simulink model "last_pressed_led"  (R2025a)
settings: Solver=FixedStepDiscrete  StartTime=0.0  StopTime=10  FixedStep=1  RelTol=1e-3
settings Model: Creator=mahij  LastModifiedBy=mahij

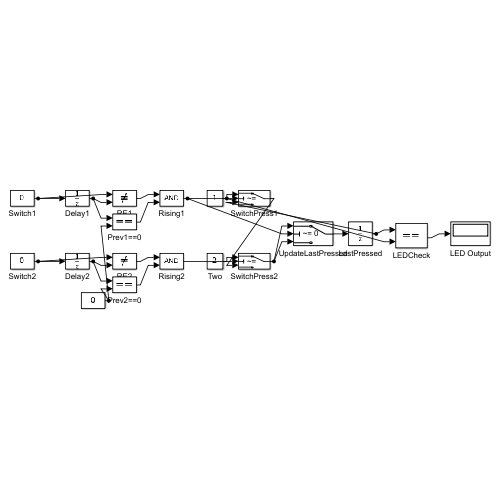
[thumbnail: Simulink's stored preview of the top-level diagram]
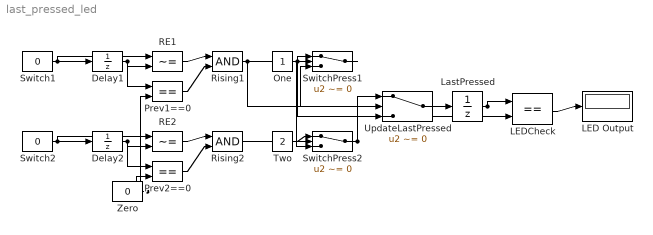
== system last_pressed_led ==
  Delay1 : UnitDelay  HasFrameUpgradeWarning=on
  Delay2 : UnitDelay  HasFrameUpgradeWarning=on
  LED Output : Display
  LEDCheck : RelationalOperator  Operator===  OutDataTypeStr=boolean  RndMeth=Simplest  InputSameDT=off
  LastPressed : UnitDelay  HasFrameUpgradeWarning=on
  One : Constant
  Prev1==0 : RelationalOperator  Operator===  OutDataTypeStr=boolean  RndMeth=Simplest  InputSameDT=off
  Prev2==0 : RelationalOperator  Operator===  OutDataTypeStr=boolean  RndMeth=Simplest  InputSameDT=off
  RE1 : RelationalOperator  Operator=~=  OutDataTypeStr=boolean  RndMeth=Simplest  InputSameDT=off
  RE2 : RelationalOperator  Operator=~=  OutDataTypeStr=boolean  RndMeth=Simplest  InputSameDT=off
  Rising1 : Logic  AllPortsSameDT=off  OutDataTypeStr=boolean
  Rising2 : Logic  AllPortsSameDT=off  OutDataTypeStr=boolean
  Switch1 : Constant  Value=0
  Switch2 : Constant  Value=0
  SwitchPress1 : Switch  Criteria=u2 ~= 0  Threshold=0.5  SaturateOnIntegerOverflow=off  InputSameDT=off
  SwitchPress2 : Switch  Criteria=u2 ~= 0  Threshold=0.5  SaturateOnIntegerOverflow=off  InputSameDT=off
  Two : Constant  Value=2
  UpdateLastPressed : Switch  Criteria=u2 ~= 0  Threshold=0.5  SaturateOnIntegerOverflow=off  InputSameDT=off
  Zero : Constant  Value=0
  wires:
  Switch1/1 -> Delay1/1, RE1/1
  Switch2/1 -> Delay2/1, RE2/1
  Delay1/1 -> RE1/2, Prev1==0/1
  Delay2/1 -> RE2/2, Prev2==0/1
  Zero/1 -> Prev1==0/2, Prev2==0/2
  RE1/1 -> Rising1/1
  Prev1==0/1 -> Rising1/2
  RE2/1 -> Rising2/1
  Prev2==0/1 -> Rising2/2
  One/1 -> SwitchPress1/1, LEDCheck/2
  Rising1/1 -> SwitchPress1/2, UpdateLastPressed/2
  LastPressed/1 -> SwitchPress1/3, LEDCheck/1
  Two/1 -> SwitchPress2/1
  Rising2/1 -> SwitchPress2/2
  SwitchPress1/1 -> SwitchPress2/3
  SwitchPress2/1 -> UpdateLastPressed/1, UpdateLastPressed/3
  UpdateLastPressed/1 -> LastPressed/1
  LEDCheck/1 -> LED Output/1
